simulink model "testing_C_functions"  (R2020b)
settings: Solver=FixedStepAuto  StartTime=0.0  StopTime=0.04  FixedStep=1e-5  RelTol=1e-3
settings Model: Creator=Kasper Laustsen  LastModifiedBy=Kasper Laustsen
settings SFSimCC: SimCustomHeaderCode="#include \"movingAvg.h\""  SimUserSources=movingAvg.c

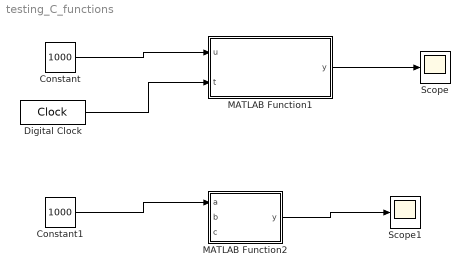
== system testing_C_functions ==
  Constant : Constant  Value=1000  SampleTime=-1
  Constant1 : Constant  Value=1000  SampleTime=-1
  Digital Clock : DigitalClock  SampleTime=1e-5
  MATLAB Function1 : MATLAB Function  TreatAsAtomicUnit=on
  MATLAB Function2 : MATLAB Function  TreatAsAtomicUnit=on
  Scope : Scope
  Scope1 : Scope
  wires:
  Constant/1 -> MATLAB Function1/1(u)
  MATLAB Function1/1(y) -> Scope/1
  Constant1/1 -> MATLAB Function2/1(a)
  MATLAB Function2/1(y) -> Scope1/1
  Digital Clock/1 -> MATLAB Function1/2(t)

== matlab function testing_C_functions/MATLAB Function2 ==
  data: a input; y output; b input; c input
function y = callingAbc_to_alphabeta(a,b,c)
coder.updateBuildInfo('addSourceFiles','abc_to_alphabeta.c');
coder.cinclude('abc_to_alphabeta.h');

y = 0.0;
y = coder.ceval('movingAvg',a,b,c);

== matlab function testing_C_functions/MATLAB Function1 ==
  data: u input; y output; t input
function y = callingMovingAvg(u,t)
coder.updateBuildInfo('addSourceFiles','movingAvg.c');
coder.cinclude('movingAvg.h');

y = 0.0;
y = coder.ceval('movingAvg',u,t);
